simulink model "planta1"  (Simulink 7.1)
settings: Solver=ode45  StartTime=0.0  StopTime=10.0  RelTol=1e-3
settings Model: Creator=ALUNO  LastModifiedBy=ALUNO

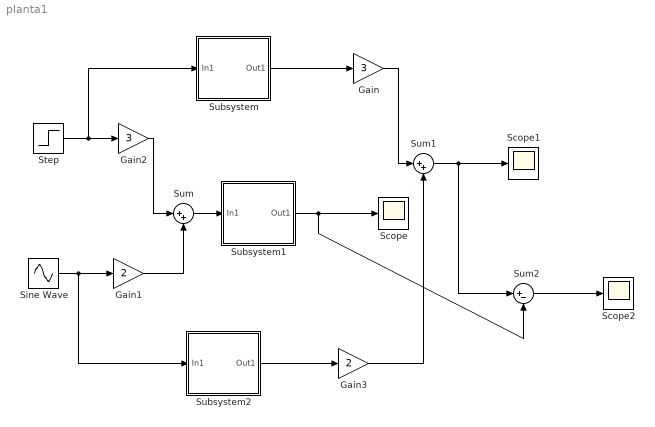
== system planta1 ==
  Gain : Gain  Gain=3  ParameterDataType=sfix(16)  ParameterScaling=2^0  OutDataType=sfix(16)  OutScaling=2^0
  Gain1 : Gain  Gain=2  ParameterDataType=sfix(16)  ParameterScaling=2^0  OutDataType=sfix(16)  OutScaling=2^0
  Gain2 : Gain  Gain=3  ParameterDataType=sfix(16)  ParameterScaling=2^0  OutDataType=sfix(16)  OutScaling=2^0
  Gain3 : Gain  Gain=2  ParameterDataType=sfix(16)  ParameterScaling=2^0  OutDataType=sfix(16)  OutScaling=2^0
  Scope : Scope
  Scope1 : Scope
  Scope2 : Scope
      settings: SaveName=ScopeData2
  Sine Wave : Sin  SampleTime=0
  Step : Step  SampleTime=0
  Subsystem : Subsystem
      mask Display: disp('Planta P1')
  Subsystem1 : Subsystem
      mask Display: disp('Planta P1')
  Subsystem2 : Subsystem
      mask Display: disp('Planta P1')
  Sum : Sum  Inputs=|++  OutDataType=sfix(16)  OutScaling=2^0
  Sum1 : Sum  Inputs=|++  OutDataType=sfix(16)  OutScaling=2^0
  Sum2 : Sum  Inputs=|+-  OutDataType=sfix(16)  OutScaling=2^0
  wires:
  Step/1 -> Gain2/1, Subsystem/1(In1)
  Sine Wave/1 -> Gain1/1, Subsystem2/1(In1)
  Subsystem2/1(Out1) -> Gain3/1
  Subsystem/1(Out1) -> Gain/1
  Gain2/1 -> Sum/1
  Gain1/1 -> Sum/2
  Sum/1 -> Subsystem1/1(In1)
  Gain/1 -> Sum1/1
  Gain3/1 -> Sum1/2
  Sum2/1 -> Scope2/1
  Sum1/1 -> Scope1/1, Sum2/1
  Subsystem1/1(Out1) -> Scope/1, Sum2/2

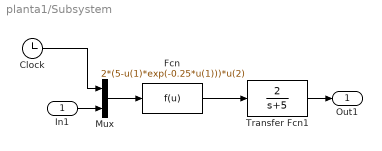
== system planta1/Subsystem ==
  In1 : Inport  OutDataType=sfix(16)  OutScaling=2^0
  Clock : Clock
      settings: Decimation=10
  Fcn : Fcn  Expr=2*(5-u(1)*exp(-0.25*u(1)))*u(2)
  Mux : Mux  Inputs=2
  Transfer Fcn1 : TransferFcn  Numerator=[2]  Denominator=[1 5]
  Out1 : Outport  OutDataType=sfix(16)  OutScaling=2^0
  wires:
  Clock/1 -> Mux/1
  Mux/1 -> Fcn/1
  Fcn/1 -> Transfer Fcn1/1
  Transfer Fcn1/1 -> Out1/1
  In1/1 -> Mux/2

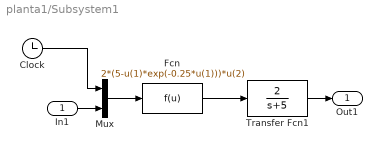
== system planta1/Subsystem1 ==
  In1 : Inport  OutDataType=sfix(16)  OutScaling=2^0
  Clock : Clock
      settings: Decimation=10
  Fcn : Fcn  Expr=2*(5-u(1)*exp(-0.25*u(1)))*u(2)
  Mux : Mux  Inputs=2
  Transfer Fcn1 : TransferFcn  Numerator=[2]  Denominator=[1 5]
  Out1 : Outport  OutDataType=sfix(16)  OutScaling=2^0
  wires:
  Clock/1 -> Mux/1
  Mux/1 -> Fcn/1
  Fcn/1 -> Transfer Fcn1/1
  Transfer Fcn1/1 -> Out1/1
  In1/1 -> Mux/2

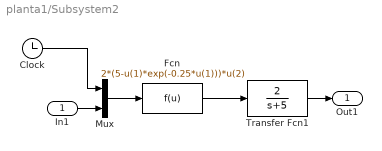
== system planta1/Subsystem2 ==
  In1 : Inport  OutDataType=sfix(16)  OutScaling=2^0
  Clock : Clock
      settings: Decimation=10
  Fcn : Fcn  Expr=2*(5-u(1)*exp(-0.25*u(1)))*u(2)
  Mux : Mux  Inputs=2
  Transfer Fcn1 : TransferFcn  Numerator=[2]  Denominator=[1 5]
  Out1 : Outport  OutDataType=sfix(16)  OutScaling=2^0
  wires:
  Clock/1 -> Mux/1
  Mux/1 -> Fcn/1
  Fcn/1 -> Transfer Fcn1/1
  Transfer Fcn1/1 -> Out1/1
  In1/1 -> Mux/2
